simulink model "sampleModel151"  (R2021b)
settings: Solver=VariableStepAuto  StartTime=0.0  StopTime=10.0  RelTol=1e-3
undefined symbols (not defined in the file or in its folder): Newton, Raphson
libraries: simulink x15, slpidlib x2
settings Model: Creator=user  LastModifiedBy=user

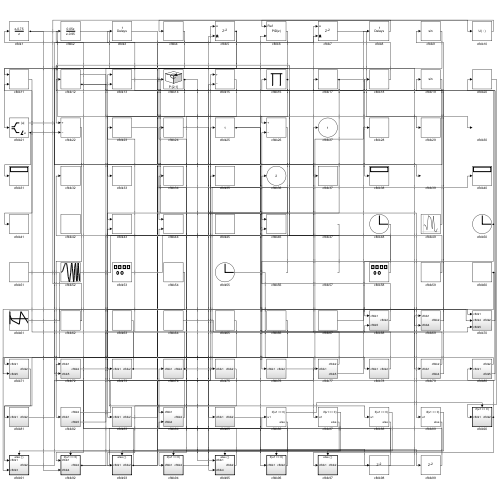
[thumbnail: Simulink's stored preview of the top-level diagram]
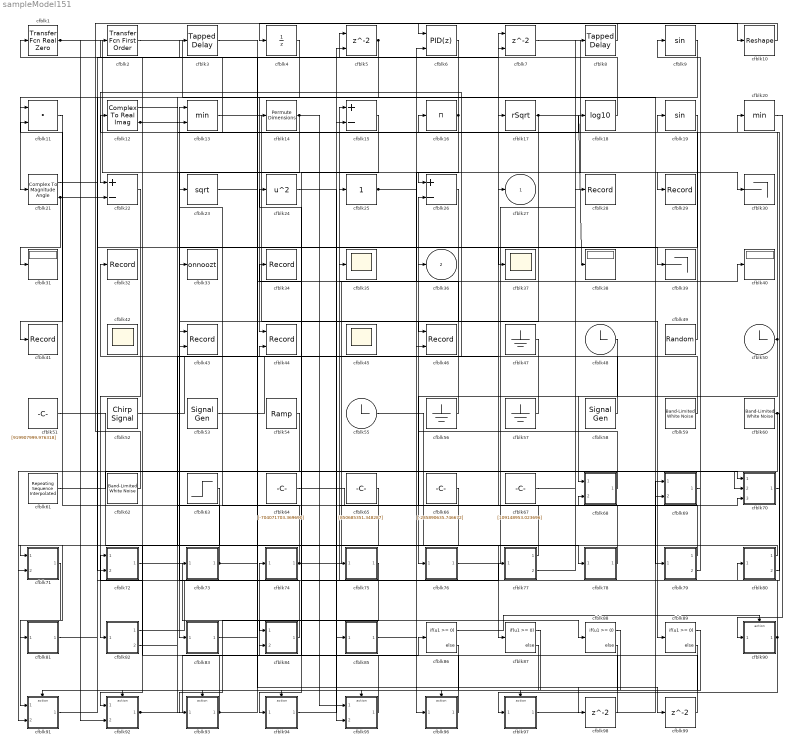
== system sampleModel151 ==
  cfblk1 : simulink/Discrete/Transfer Fcn Real Zero  ZeroZ=0.75  ICPrevInput=0.0  DoSatur=off
      settings: SourceProductBaseCode=SL
  cfblk10 : Reshape
  cfblk11 : DotProduct  InputSameDT=on  OutDataTypeStr=Inherit: Inherit via internal rule
  cfblk12 : ComplexToRealImag
  cfblk13 : MinMax  Inputs=2
  cfblk14 : PermuteDimensions
  cfblk15 : Sum  Inputs=+-
  cfblk16 : Product  Inputs=*
  cfblk17 : Sqrt  Operator=rSqrt  AlgorithmType=Newton-Raphson  SaturateOnIntegerOverflow=on
  cfblk18 : Math  Operator=log10  SaturateOnIntegerOverflow=on
  cfblk19 : Trigonometry
  cfblk2 : simulink/Discrete/Transfer Fcn First Order  PoleZ=0.95  ICPrevOutput=0.0  DoSatur=off
  cfblk20 : MinMax
  cfblk21 : ComplexToMagnitudeAngle
  cfblk22 : Sum  Inputs=+-
  cfblk23 : Sqrt  SaturateOnIntegerOverflow=on
  cfblk24 : Math  Operator=square  SaturateOnIntegerOverflow=on
  cfblk25 : simulink/Math Operations/Slider Gain  gain=1  low=0  high=2
  cfblk26 : Sum  Inputs=+-
  cfblk28 : Record  FileSettingsInternal="{\"entries\":[{\"content\":{\"excelSettings\":{\"content\":{},\"type\":\"Streamout.ExcelSettings\"}},\"type\":\"Streamout.FileSettingStorage\",\"uuid\":\"16329020-b7b2-48e2-bef7-29498af02094\"}],\"packageUris\":[\"http://schema.mathworks.com/mf0/streamout_blocks/R2020a\"],\"version\":\"1.0\"}"  SignalsInternal="{\"entries\":[{\"content\":{\"signals\":[{\"content\":{\"blockPath\":[\"sampleModel151/cfblk28\"],\"channel\":[],\"dimensions\":[1],\"domain\":\"sampleModel151/cfblk28\",\"lineColor\":\"#fe330a\",\"plots\":[1],\"port\":1,\"sid\":[\"\"],\"signalID\":5566,\"signalName\":\"cfblk77:2\"},\"type\":\"RecordBlkView.Signal\",\"uuid\":\"cbec37e1-0653-4d3b-993b-30f071d7b7c2\"}]},\"type\":\"RecordBlkView.InputSignals\",\"uuid\":\"1aea9fb2-e907-4a06-aea3-794993e5d476\"}],\"packageUris\":[\"http://schema.mathworks.com/mf0/streamout_blocks/R2020a\"],\"version\":\"1.0\"}"  VisualizationBindings="{\"sparklinesplugin\":{\"info\":[{\"bindingParametersList\":[],\"subplotID\":1}]}}"
  cfblk29 : Record  FileSettingsInternal="{\"entries\":[{\"content\":{\"excelSettings\":{\"content\":{},\"type\":\"Streamout.ExcelSettings\"}},\"type\":\"Streamout.FileSettingStorage\",\"uuid\":\"ad175cd4-5bed-4ac1-be59-b4bcf34f1e7c\"}],\"packageUris\":[\"http://schema.mathworks.com/mf0/streamout_blocks/R2020a\"],\"version\":\"1.0\"}"  SignalsInternal="{\"entries\":[{\"content\":{\"signals\":[{\"content\":{\"blockPath\":[\"sampleModel151/cfblk29\"],\"channel\":[],\"dimensions\":[1,1],\"domain\":\"sampleModel151/cfblk29\",\"lineColor\":\"#22b573\",\"plots\":[1],\"port\":1,\"sid\":[\"\"],\"signalID\":5570,\"signalName\":\"cfblk7\"},\"type\":\"RecordBlkView.Signal\",\"uuid\":\"59788e8c-d7b2-4cd3-8900-8817d59cbc28\"}]},\"type\":\"RecordBlkView.InputSignals\",\"uuid\":\"d411062e-e278-425d-97f2-c320e6c0c2a0\"}],\"packageUris\":[\"http://schema.mathworks.com/mf0/streamout_blocks/R2020a\"],\"version\":\"1.0\"}"  VisualizationBindings="{\"sparklinesplugin\":{\"info\":[{\"bindingParametersList\":[],\"subplotID\":1}]}}"
  cfblk3 : simulink/Discrete/Tapped Delay  vinit=0.0  samptime=-1  NumDelays=1  DelayOrder=Oldest  includeCurrent=off
  cfblk30 : Terminator
  cfblk31 : Display
  cfblk32 : Record  FileSettingsInternal="{\"entries\":[{\"content\":{\"excelSettings\":{\"content\":{},\"type\":\"Streamout.ExcelSettings\"}},\"type\":\"Streamout.FileSettingStorage\",\"uuid\":\"e17f7bcd-ee65-47d5-ad36-393b5ddf6025\"}],\"packageUris\":[\"http://schema.mathworks.com/mf0/streamout_blocks/R2020a\"],\"version\":\"1.0\"}"  SignalsInternal="{\"entries\":[{\"content\":{\"signals\":[{\"content\":{\"blockPath\":[\"sampleModel151/cfblk32\"],\"channel\":[],\"dimensions\":[1],\"domain\":\"sampleModel151/cfblk32\",\"lineColor\":\"#139fff\",\"plots\":[1],\"port\":1,\"sid\":[\"\"],\"signalID\":5602,\"signalName\":\"cfblk59\"},\"type\":\"RecordBlkView.Signal\",\"uuid\":\"9c12727e-2af6-4ba1-9340-e75212aef403\"}]},\"type\":\"RecordBlkView.InputSignals\",\"uuid\":\"08633602-5334-4035-af5c-359580bce636\"}],\"packageUris\":[\"http://schema.mathworks.com/mf0/streamout_blocks/R2020a\"],\"version\":\"1.0\"}"  VisualizationBindings="{\"sparklinesplugin\":{\"info\":[{\"bindingParametersList\":[],\"subplotID\":1}]}}"
  cfblk33 : ToWorkspace  VariableName=onnoozt  SaveFormat=Timeseries  SampleTime=-1
  cfblk34 : Record  FileSettingsInternal="{\"entries\":[{\"content\":{\"excelSettings\":{\"content\":{},\"type\":\"Streamout.ExcelSettings\"}},\"type\":\"Streamout.FileSettingStorage\",\"uuid\":\"80bf3479-7660-47d1-b758-6739f5e518e5\"}],\"packageUris\":[\"http://schema.mathworks.com/mf0/streamout_blocks/R2020a\"],\"version\":\"1.0\"}"  SignalsInternal="{\"entries\":[{\"content\":{\"signals\":[{\"content\":{\"blockPath\":[\"sampleModel151/cfblk34\"],\"channel\":[],\"dimensions\":[1],\"domain\":\"sampleModel151/cfblk34\",\"lineColor\":\"#0072bd\",\"plots\":[1],\"port\":1,\"sid\":[\"\"],\"signalID\":5574,\"signalName\":\"cfblk90\"},\"type\":\"RecordBlkView.Signal\",\"uuid\":\"52cf2cfa-6272-4b00-98cf-892733082b01\"}]},\"type\":\"RecordBlkView.InputSignals\",\"uuid\":\"b0825b05-81fc-4d9b-a675-fd277561146e\"}],\"packageUris\":[\"http://schema.mathworks.com/mf0/streamout_blocks/R2020a\"],\"version\":\"1.0\"}"  VisualizationBindings="{\"sparklinesplugin\":{\"info\":[{\"bindingParametersList\":[],\"subplotID\":1}]}}"
  cfblk{35,37,42,45} (4 alike) : Scope
      cfblk42 settings: Floating=on
      cfblk45 settings: Floating=on
  cfblk38 : Display
  cfblk39 : Terminator
  cfblk4 : UnitDelay  HasFrameUpgradeWarning=on
  cfblk40 : Display
  cfblk41 : Record  FileSettingsInternal="{\"entries\":[{\"content\":{\"excelSettings\":{\"content\":{},\"type\":\"Streamout.ExcelSettings\"}},\"type\":\"Streamout.FileSettingStorage\",\"uuid\":\"e783f573-5e51-434e-8b39-352c88833e99\"}],\"packageUris\":[\"http://schema.mathworks.com/mf0/streamout_blocks/R2020a\"],\"version\":\"1.0\"}"  SignalsInternal="{\"entries\":[{\"content\":{\"signals\":[{\"content\":{\"blockPath\":[\"sampleModel151/cfblk41\"],\"channel\":[],\"dimensions\":[1],\"domain\":\"sampleModel151/cfblk41\",\"lineColor\":\"#d95319\",\"plots\":[1],\"port\":1,\"sid\":[\"\"],\"signalID\":5578,\"signalName\":\"cfblk11\"},\"type\":\"RecordBlkView.Signal\",\"uuid\":\"9378f9bf-08aa-425a-ab1e-6e49c199abac\"}]},\"type\":\"RecordBlkView.InputSignals\",\"uuid\":\"4020c576-885d-4cd6-9814-44353d409ce4\"}],\"packageUris\":[\"http://schema.mathworks.com/mf0/streamout_blocks/R2020a\"],\"version\":\"1.0\"}"  VisualizationBindings="{\"sparklinesplugin\":{\"info\":[{\"bindingParametersList\":[],\"subplotID\":1}]}}"
  cfblk43 : Record  FileSettingsInternal="{\"entries\":[{\"content\":{\"excelSettings\":{\"content\":{},\"type\":\"Streamout.ExcelSettings\"}},\"type\":\"Streamout.FileSettingStorage\",\"uuid\":\"0c75c6a2-1ebc-4dbd-9707-8aa0bfb7056d\"}],\"packageUris\":[\"http://schema.mathworks.com/mf0/streamout_blocks/R2020a\"],\"version\":\"1.0\"}"  Layout=[1 1]  SignalsInternal="{\"entries\":[{\"content\":{\"signals\":[{\"content\":{\"blockPath\":[\"sampleModel151/cfblk43\"],\"channel\":[],\"dimensions\":[1],\"domain\":\"sampleModel151/cfblk43\",\"lineColor\":\"#a2142f\",\"plots\":[1],\"port\":1,\"sid\":[\"\"],\"signalID\":5582,\"signalName\":\"cfblk26\"},\"type\":\"RecordBlkView.Signal\",\"uuid\":\"05fc9d93-6de0-4f23-9265-e6d9e86d6584\"},{\"content\":{\"blockPath\":[\"sampleModel151/cfblk43\"],\"channel\":[],\"dimensions\":[1],\"domain\":\"sampleModel151/cfblk43\",\"lineColor\":\"#139fff\",\"plots\":[1],\"port\":2,\"sid\":[\"\"],\"signalID\":5606,\"signalName\":\"cfblk47\"},\"type\":\"RecordBlkView.Signal\",\"uuid\":\"81c749a0-ca2e-451c-aa8b-75db0fa4dd54\"}]},\"type\":\"RecordBlkView.InputSignals\",\"uuid\":\"aefd6379-81b4-49ca-99cc-edc691e51c33\"}],\"packageUris\":[\"http://schema.mathworks.com/mf0/streamout_blocks/R2020a\"],\"version\":\"1.0\"}"  VisualizationBindings="{\"xyplotplugin\":{\"info\":[{\"series\":[{\"bindingParametersList\":[{\"parameter\":\"X-Axis\",\"signalID\":5582,\"signalName\":\"cfblk26\"},{\"parameter\":\"Y-Axis\",\"signalID\":5606,\"signalName\":\"cfblk47\"}],\"seriesID\":51947}],\"subplotID\":1}]}}"  CompatibilityTag=XY
  cfblk44 : Record  FileSettingsInternal="{\"entries\":[{\"content\":{\"excelSettings\":{\"content\":{},\"type\":\"Streamout.ExcelSettings\"}},\"type\":\"Streamout.FileSettingStorage\",\"uuid\":\"e408540b-f554-4ccd-875e-bc098b567ff3\"}],\"packageUris\":[\"http://schema.mathworks.com/mf0/streamout_blocks/R2020a\"],\"version\":\"1.0\"}"  Layout=[1 1]  SignalsInternal="{\"entries\":[{\"content\":{\"signals\":[{\"content\":{\"blockPath\":[\"sampleModel151/cfblk44\"],\"channel\":[],\"dimensions\":[1],\"domain\":\"sampleModel151/cfblk44\",\"lineColor\":\"#a2142f\",\"plots\":[1],\"port\":1,\"sid\":[\"\"],\"signalID\":5586,\"signalName\":\"cfblk16\"},\"type\":\"RecordBlkView.Signal\",\"uuid\":\"6af45d05-4fcc-41dc-a0e5-1353e5ef8c24\"},{\"content\":{\"blockPath\":[\"sampleModel151/cfblk44\"],\"channel\":[],\"dimensions\":[1],\"domain\":\"sampleModel151/cfblk44\",\"lineColor\":\"#139fff\",\"plots\":[1],\"port\":2,\"sid\":[\"\"],\"signalID\":5590,\"signalName\":\"cfblk82:2\"},\"type\":\"RecordBlkView.Signal\",\"uuid\":\"fc406fd3-a582-4b99-9ff1-c8c34bae7090\"}]},\"type\":\"RecordBlkView.InputSignals\",\"uuid\":\"f27d2fd3-ba63-49dc-9794-1473fbe6710d\"}],\"packageUris\":[\"http://schema.mathworks.com/mf0/streamout_blocks/R2020a\"],\"version\":\"1.0\"}"  VisualizationBindings="{\"xyplotplugin\":{\"info\":[{\"series\":[{\"bindingParametersList\":[{\"parameter\":\"X-Axis\",\"signalID\":5586,\"signalName\":\"cfblk16\"},{\"parameter\":\"Y-Axis\",\"signalID\":5590,\"signalName\":\"cfblk82:2\"}],\"seriesID\":36672}],\"subplotID\":1}]}}"  CompatibilityTag=XY
  cfblk46 : Record  FileSettingsInternal="{\"entries\":[{\"content\":{\"excelSettings\":{\"content\":{},\"type\":\"Streamout.ExcelSettings\"}},\"type\":\"Streamout.FileSettingStorage\",\"uuid\":\"872aefc3-b221-4a71-9802-efcb06a78721\"}],\"packageUris\":[\"http://schema.mathworks.com/mf0/streamout_blocks/R2020a\"],\"version\":\"1.0\"}"  Layout=[1 1]  SignalsInternal="{\"entries\":[{\"content\":{\"signals\":[{\"content\":{\"blockPath\":[\"sampleModel151/cfblk46\"],\"channel\":[],\"dimensions\":[1],\"domain\":\"sampleModel151/cfblk46\",\"lineColor\":\"#a2142f\",\"plots\":[1],\"port\":1,\"sid\":[\"\"],\"signalID\":5594,\"signalName\":\"cfblk24\"},\"type\":\"RecordBlkView.Signal\",\"uuid\":\"f73d4481-3b9c-43d6-816d-b610603f159a\"},{\"content\":{\"blockPath\":[\"sampleModel151/cfblk46\"],\"channel\":[],\"dimensions\":[1],\"domain\":\"sampleModel151/cfblk46\",\"lineColor\":\"#139fff\",\"plots\":[1],\"port\":2,\"sid\":[\"\"],\"signalID\":5598,\"signalName\":\"cfblk16\"},\"type\":\"RecordBlkView.Signal\",\"uuid\":\"61bf5f49-bdad-4a1e-a78b-57c9270c8f12\"}]},\"type\":\"RecordBlkView.InputSignals\",\"uuid\":\"eca14434-e9e9-4071-bd11-9bcd73b8db11\"}],\"packageUris\":[\"http://schema.mathworks.com/mf0/streamout_blocks/R2020a\"],\"version\":\"1.0\"}"  VisualizationBindings="{\"xyplotplugin\":{\"info\":[{\"series\":[{\"bindingParametersList\":[{\"parameter\":\"X-Axis\",\"signalID\":5594,\"signalName\":\"cfblk24\"},{\"parameter\":\"Y-Axis\",\"signalID\":5598,\"signalName\":\"cfblk16\"}],\"seriesID\":29055}],\"subplotID\":1}]}}"  CompatibilityTag=XY
  cfblk47 : Ground
  cfblk48 : Clock
  cfblk49 : RandomNumber  Mean=[30540.773261]  Variance=[36221.773960]  Seed=[260701924.000000]  SampleTime=0.1
  cfblk5 : Delay  ShowEnablePort=on  SampleTime=1
      settings: InputPortMap=u0,e6
  cfblk50 : Clock
  cfblk51 : Constant  Value=[919907999.976318]  SampleTime=1
  cfblk52 : simulink/Sources/Chirp Signal  f1=[-683339794.347448]  T=[-526882344.998948]  f2=[43752890.467036]
  cfblk53 : SignalGenerator  WaveForm=sawtooth  Amplitude=[-680922363.172468]
  cfblk54 : simulink/Sources/Ramp  slope=[1986.058143]  start=[19.480931]  InitialOutput=[55276.021662]
  cfblk55 : Clock
  cfblk56 : Ground
  cfblk57 : Ground
  cfblk58 : SignalGenerator  WaveForm=sawtooth  Amplitude=[-424760600.039455]
  cfblk59 : simulink/Sources/Band-Limited White Noise  Cov=[1215861451.663982]  Ts=0.1  seed=[1365901163.000000]
  cfblk6 : slpidlib/PID Controller (2DOF)  Controller=PID  Form=Parallel  TimeDomain=Discrete-time  UseExternalTs=off  SampleTime=1  IntegratorMethod=Forward Euler  FilterMethod=Forward Euler  ControllerParametersSource=internal  P=1  I=1  D=0  UseFilter=on  N=100  b=1  c=1  TunerSelectOption=Transfer Function Based (PID Tuner App)  InitialConditionSource=internal  InitialConditionForIntegrator=0  InitialConditionForFilter=0  DifferentiatorICPrevScaledInput=0  ExternalReset=none  TrackingMode=off  Kt=1  LimitOutput=off  SatLimitsSource=internal  UpperSaturationLimit=inf  LowerSaturationLimit=-inf  LinearizeAsGain=off  AntiWindupMode=none  Kb=1  POutMin=[]  POutMax=[]  IOutMin=[]  IOutMax=[]  DOutMin=[]  DOutMax=[]  NOutMin=[]  NOutMax=[]  bOutMin=[]  bOutMax=[]  cOutMin=[]  cOutMax=[]  SumOutMin=[]  SumOutMax=[]  SaturationOutMin=[]  SaturationOutMax=[]  PParamMin=[]  PParamMax=[]  IParamMin=[]  IParamMax=[]  DParamMin=[]  DParamMax=[]  NParamMin=[]  NParamMax=[]  bParamMin=[]  bParamMax=[]  cParamMin=[]  cParamMax=[]  KbParamMin=[]  KbParamMax=[]  KtParamMin=[]  KtParamMax=[]  KbOutMin=[]  KbOutMax=[]  KtOutMin=[]  KtOutMax=[]  IntegratorOutMin=[]  IntegratorOutMax=[]  FilterOutMin=[]  FilterOutMax=[]  SumI1OutMin=[]  SumI1OutMax=[]  SumI2OutMin=[]  SumI2OutMax=[]  SumI3OutMin=[]  SumI3OutMax=[]  SumI4OutMin=[]  SumI4OutMax=[]  SumDOutMin=[]  SumDOutMax=[]  Sum1OutMin=[]  Sum1OutMax=[]  Sum2OutMin=[]  Sum2OutMax=[]  Sum3OutMin=[]  Sum3OutMax=[]  DifferentiatorOutMin=[]  DifferentiatorOutMax=[]  FilterDiffOutCoefMin=[]  FilterDiffOutCoefMax=[]  ReciprocalOutMin=[]  ReciprocalOutMax=[]  SumDenOutMin=[]  SumDenOutMax=[]  SumNumOutMin=[]  SumNumOutMax=[]  DivideOutMin=[]  DivideOutMax=[]  UdiffTsProdOutMin=[]  UdiffTsProdOutMax=[]  NTsProdOutMin=[]  NTsProdOutMax=[]  UintegralTsProdOutMin=[]  UintegralTsProdOutMax=[]  UngainTsProdOutMin=[]  UngainTsProdOutMax=[]  IntegratorContinuousStateAttributes=''  IntegratorStateMustResolveToSignalObject=off  IntegratorRTWStateStorageClass=Auto  FilterContinuousStateAttributes=''  FilterStateMustResolveToSignalObject=off  FilterRTWStateStorageClass=Auto  ParallelPVariant=InternalParameters  IdealPVariant=Disabled  IVariant=InternalParameters  DVariant=InternalParameters  bVariant=InternalParameters  cVariant=InternalParameters  IntegratorVariant=Discrete  SatVariant=Disabled  AWVariant=Passthrough  PCopyVariant=Disabled  TRVariant=Disabled  FdbkBlocksVariant=Forward  IdealPFdbkVariant=Disabled  SatFdbkVariant=Disabled  DerivativeFilterVariant=ForwardEulerFilter  NVariant=InternalParameters  NCopyVariant=Disabled  FilterICVariant=InternalICsFilter  IntegratorICVariant=InternalICs  ExternalResetVariant=Disabled  TRSumVariant=Passthrough  SumFdbkVariant=Disabled  SumVariant=Sum_PID  TsampFilterVariant=InternalTs  TsampNgainVariant=Passthrough  TsampIntegralVariant=Passthrough  ExternalSaturationOutDataTypeStr=Inherit: Same as second input
      settings: SourceProductBaseCode=SL
  cfblk60 : simulink/Sources/Band-Limited White Noise  Cov=[7735132577.981955]  Ts=0.1  seed=[9624433011.000000]
  cfblk61 : simulink/Sources/Repeating Sequence Interpolated  OutValues=[321209929.759004, -164411513.665843, -521363815.949086, 697235986.617966, -429595361.275155]  TimeValues=[0 0.1 0.5 0.6 1].'  LookUpMeth=Use Input Below  tsamp=0.01  OutMin=[]  OutMax=[]  OutDataTypeStr=double  OutputDataTypeScalingMode=double  OutDataType=fixdt(0,8)  OutScaling=2^-10
  cfblk62 : simulink/Sources/Band-Limited White Noise  Cov=[8435027631.011647]  Ts=0.1  seed=[5841098064.000000]
  cfblk63 : Step  Time=[4.000000]  Before=[11276169.714796]  After=[23174660.640238]  SampleTime=0
  cfblk64 : Constant  Value=[-704071703.369690]  SampleTime=1
  cfblk65 : Constant  Value=[850685351.348287]  SampleTime=1
  cfblk66 : Constant  Value=[-285890635.746672]  SampleTime=1
  cfblk67 : Constant  Value=[109148953.023696]  SampleTime=1
  cfblk68 : Subsystem
  cfblk69 : Subsystem
  cfblk7 : Delay  ShowEnablePort=on  SampleTime=1
      settings: InputPortMap=u0,e6
  cfblk70 : Subsystem
  cfblk71 : Subsystem
  cfblk72 : Subsystem
  cfblk73 : Subsystem
  cfblk74 : Subsystem
  cfblk75 : Subsystem
  cfblk76 : Subsystem
  cfblk77 : Subsystem
  cfblk78 : Subsystem
  cfblk79 : Subsystem
  cfblk8 : simulink/Discrete/Tapped Delay  vinit=0.0  samptime=-1  NumDelays=1  DelayOrder=Oldest  includeCurrent=off
  cfblk80 : Subsystem
  cfblk81 : Subsystem
  cfblk82 : Subsystem
  cfblk83 : Subsystem
  cfblk84 : Subsystem
  cfblk85 : Subsystem
  cfblk{86..89} (4 alike) : If  IfExpression=u1 >= 0  SampleTime=1
  cfblk9 : Trigonometry
  cfblk90 : Subsystem  TreatAsAtomicUnit=on
  cfblk91 : Subsystem  TreatAsAtomicUnit=on
  cfblk92 : Subsystem  TreatAsAtomicUnit=on
  cfblk93 : Subsystem  TreatAsAtomicUnit=on
  cfblk94 : Subsystem  TreatAsAtomicUnit=on
  cfblk95 : Subsystem  TreatAsAtomicUnit=on
  cfblk96 : Subsystem  TreatAsAtomicUnit=on
  cfblk97 : Subsystem  TreatAsAtomicUnit=on
  cfblk98 : Delay  SampleTime=1
  cfblk99 : Delay  SampleTime=1
  cfblk27 : Outport
  cfblk36 : Outport  Port=2
  wires:
  cfblk79/1(cfblk2) -> cfblk15/1
  cfblk84/1(cfblk2) -> cfblk13/1
  cfblk16/1 -> cfblk44/1, cfblk46/2
  cfblk92/1(cfblk2) -> cfblk86/1, cfblk70/3(cfblk5)
  cfblk57/1 -> cfblk22/1
  cfblk59/1 -> cfblk32/1
  cfblk85/1(cfblk2) -> cfblk96/1(cfblk1)
  cfblk15/1 -> cfblk94/1(cfblk1)
  cfblk69/1(cfblk2) -> cfblk9/1
  cfblk14/1 -> cfblk83/1(cfblk1), cfblk95/1(cfblk1)
  cfblk80/1(cfblk2) -> cfblk71/1(cfblk1)
  cfblk75/1(cfblk2) -> cfblk93/1(cfblk1)
  cfblk62/1 -> cfblk10/1
  cfblk82/1(cfblk2) -> cfblk25/1
  cfblk22/1 -> cfblk82/1(cfblk1)
  cfblk60/1 -> cfblk80/1(cfblk1), cfblk91/2(cfblk3)
  cfblk65/1 -> cfblk71/2(cfblk5)
  cfblk13/1 -> cfblk89/1
  cfblk93/1(cfblk2) -> cfblk5/1, cfblk40/1, cfblk72/1(cfblk1)
  cfblk77/1(cfblk2) -> cfblk7/1
  cfblk19/1 -> cfblk33/1
  cfblk50/1 -> cfblk68/1(cfblk1), cfblk3/1
  cfblk6/1 -> cfblk21/1
  cfblk9/1 -> cfblk11/1
  cfblk67/1 -> cfblk70/1(cfblk1)
  cfblk66/1 -> cfblk92/1(cfblk1)
  cfblk48/1 -> cfblk76/1(cfblk1)
  cfblk96/1(cfblk2) -> cfblk74/1(cfblk1)
  cfblk1/1 -> cfblk26/1, cfblk92/2(cfblk4)
  cfblk8/1 -> cfblk6/1
  cfblk18/1 -> cfblk1/1
  cfblk20/1 -> cfblk90/1(cfblk1)
  cfblk56/1 -> cfblk35/1
  cfblk90/1(cfblk2) -> cfblk97/1(cfblk1), cfblk34/1
  cfblk53/1 -> cfblk27/1
  cfblk91/1(cfblk2) -> cfblk7/2
  cfblk26/1 -> cfblk43/1
  cfblk21/1 -> cfblk39/1
  cfblk4/1 -> cfblk13/2
  cfblk71/1(cfblk2) -> cfblk91/1(cfblk1)
  cfblk78/1(cfblk2) -> cfblk26/2
  cfblk94/1(cfblk2) -> cfblk5/2
  cfblk55/1 -> cfblk87/1
  cfblk74/1(cfblk2) -> cfblk6/2, cfblk23/1
  cfblk10/1 -> cfblk4/1
  cfblk52/1 -> cfblk15/2
  cfblk80/2(cfblk5) -> cfblk12/1
  cfblk72/1(cfblk2) -> cfblk84/1(cfblk1)
  cfblk12/1 -> cfblk78/1(cfblk1)
  cfblk11/1 -> cfblk41/1
  cfblk97/1(cfblk2) -> cfblk69/1(cfblk1)
  cfblk25/1 -> cfblk69/2(cfblk4), cfblk98/1
  cfblk68/1(cfblk2) -> cfblk36/1
  cfblk24/1 -> cfblk46/1
  cfblk79/2(cfblk4) -> cfblk17/1
  cfblk5/1 -> cfblk22/2, cfblk72/2(cfblk5)
  cfblk2/1 -> cfblk79/1(cfblk1)
  cfblk54/1 -> cfblk73/1(cfblk1)
  cfblk81/1(cfblk2) -> cfblk75/1(cfblk1)
  cfblk64/1 -> cfblk68/2(cfblk5)
  cfblk47/1 -> cfblk43/2
  cfblk49/1 -> cfblk19/1
  cfblk7/1 -> cfblk29/1
  cfblk12/2 -> cfblk30/1, cfblk18/1
  cfblk3/1 -> cfblk88/1
  cfblk58/1 -> cfblk16/1
  cfblk17/1 -> cfblk38/1, cfblk95/2(cfblk4)
  cfblk73/1(cfblk2) -> cfblk14/1, cfblk11/2
  cfblk77/2(cfblk5) -> cfblk28/1
  cfblk76/1(cfblk2) -> cfblk8/1
  cfblk63/1 -> cfblk81/1(cfblk1)
  cfblk51/1 -> cfblk85/1(cfblk1)
  cfblk61/1 -> cfblk70/2(cfblk4)
  cfblk82/2(cfblk5) -> cfblk44/2
  cfblk95/1(cfblk2) -> cfblk24/1
  cfblk21/2 -> cfblk37/1, cfblk31/1
  cfblk70/1(cfblk2) -> cfblk20/1
  cfblk83/1(cfblk2) -> cfblk77/1(cfblk1)
  cfblk86/1 -> cfblk90/Action
  cfblk86/2 -> cfblk91/Action
  cfblk87/1 -> cfblk92/Action
  cfblk87/2 -> cfblk93/Action
  cfblk88/1 -> cfblk94/Action
  cfblk88/2 -> cfblk95/Action
  cfblk89/1 -> cfblk96/Action
  cfblk89/2 -> cfblk97/Action
  cfblk98/1 -> cfblk2/1
  cfblk23/1 -> cfblk99/1
  cfblk99/1 -> cfblk84/2(cfblk4)

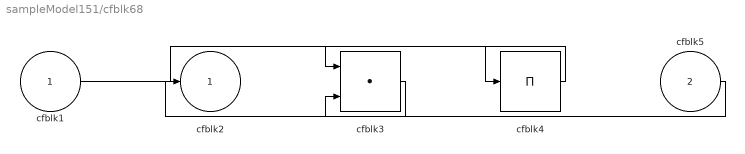
== system sampleModel151/cfblk68 ==
  cfblk1 : Inport
  cfblk5 : Inport  Port=2
  cfblk3 : DotProduct  InputSameDT=on  OutDataTypeStr=Inherit: Inherit via internal rule
  cfblk4 : Product  Inputs=*
  cfblk2 : Outport
  wires:
  cfblk1/1 -> cfblk4/1
  cfblk3/1 -> cfblk2/1
  cfblk4/1 -> cfblk3/1
  cfblk5/1 -> cfblk3/2

== system sampleModel151/cfblk69 ==
  cfblk1 : Inport
  cfblk4 : Inport  Port=2
  cfblk3 : simulink/Discrete/Difference  ICPrevInput=0.0  OutMin=[]  OutMax=[]  OutDataTypeStr=Inherit: Inherit via back propagation  OutDataType=fixdt(1, 16)  OutScaling=2^-10  DoSatur=off
  cfblk2 : Outport
  wires:
  cfblk1/1 -> cfblk3/1
  cfblk4/1 -> cfblk2/1

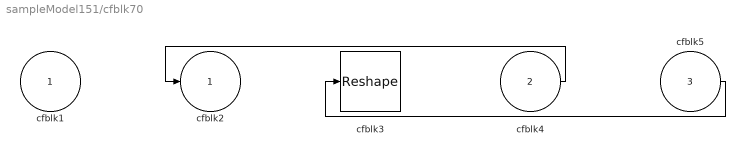
== system sampleModel151/cfblk70 ==
  cfblk1 : Inport
  cfblk4 : Inport  Port=2
  cfblk5 : Inport  Port=3
  cfblk3 : Reshape
  cfblk2 : Outport
  wires:
  cfblk4/1 -> cfblk2/1
  cfblk5/1 -> cfblk3/1

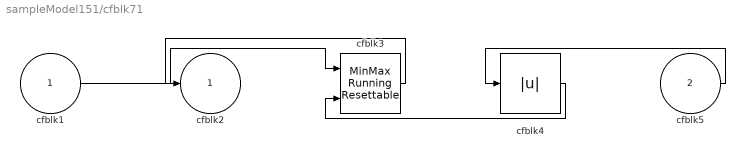
== system sampleModel151/cfblk71 ==
  cfblk1 : Inport
  cfblk5 : Inport  Port=2
  cfblk3 : simulink/Math Operations/MinMax Running Resettable  Function=min  vinit=0.0
  cfblk4 : Abs
  cfblk2 : Outport
  wires:
  cfblk5/1 -> cfblk4/1
  cfblk1/1 -> cfblk3/1
  cfblk4/1 -> cfblk3/2
  cfblk3/1 -> cfblk2/1

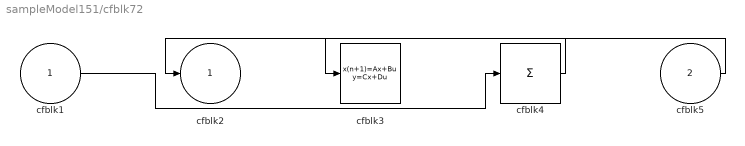
== system sampleModel151/cfblk72 ==
  cfblk1 : Inport
  cfblk5 : Inport  Port=2
  cfblk3 : DiscreteStateSpace
  cfblk4 : Sum  Inputs=+
  cfblk2 : Outport
  wires:
  cfblk5/1 -> cfblk2/1
  cfblk1/1 -> cfblk4/1
  cfblk4/1 -> cfblk3/1

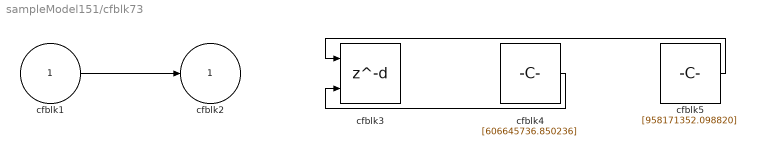
== system sampleModel151/cfblk73 ==
  cfblk1 : Inport
  cfblk3 : Delay  DelayLengthSource=Input port  SampleTime=1
      settings: InputPortMap=u0,p1
  cfblk4 : Constant  Value=[606645736.850236]  SampleTime=1
  cfblk5 : Constant  Value=[958171352.098820]  SampleTime=1
  cfblk2 : Outport
  wires:
  cfblk1/1 -> cfblk2/1
  cfblk5/1 -> cfblk3/1
  cfblk4/1 -> cfblk3/2

== system sampleModel151/cfblk74 ==
  cfblk1 : Inport
  cfblk3 : Sum  Inputs=+
  cfblk4 : Sin  TimeSource=Use external signal  SampleTime=0
  cfblk2 : Outport
  wires:
  cfblk1/1 -> cfblk3/1
  cfblk4/1 -> cfblk2/1
  cfblk3/1 -> cfblk4/1

== system sampleModel151/cfblk75 ==
  cfblk1 : Inport
  cfblk3 : Rounding
  cfblk4 : UnaryMinus
  cfblk2 : Outport
  wires:
  cfblk1/1 -> cfblk4/1
  cfblk4/1 -> cfblk3/1
  cfblk3/1 -> cfblk2/1

== system sampleModel151/cfblk76 ==
  cfblk1 : Inport
  cfblk3 : Constant  Value=[-952970532.415323]  SampleTime=1
  cfblk2 : Outport
  wires:
  cfblk3/1 -> cfblk2/1

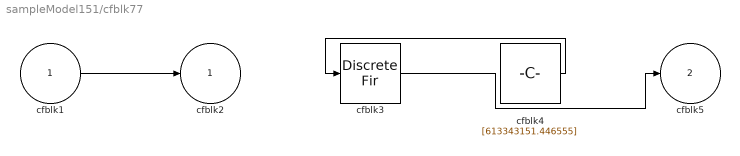
== system sampleModel151/cfblk77 ==
  cfblk1 : Inport
  cfblk3 : DiscreteFir  SampleTime=1
  cfblk4 : Constant  Value=[613343151.446555]  SampleTime=1
  cfblk2 : Outport
  cfblk5 : Outport  Port=2
  wires:
  cfblk4/1 -> cfblk3/1
  cfblk3/1 -> cfblk5/1
  cfblk1/1 -> cfblk2/1

== system sampleModel151/cfblk78 ==
  cfblk1 : Inport
  cfblk3 : DotProduct  InputSameDT=on  OutDataTypeStr=Inherit: Inherit via internal rule
  cfblk2 : Outport
  wires:
  cfblk3/1 -> cfblk2/1
  cfblk1/1 -> cfblk3/1, cfblk3/2

== system sampleModel151/cfblk79 ==
  cfblk1 : Inport
  cfblk3 : DiscreteFir  SampleTime=1
  cfblk2 : Outport
  cfblk4 : Outport  Port=2
  wires:
  cfblk1/1 -> cfblk2/1, cfblk3/1
  cfblk3/1 -> cfblk4/1

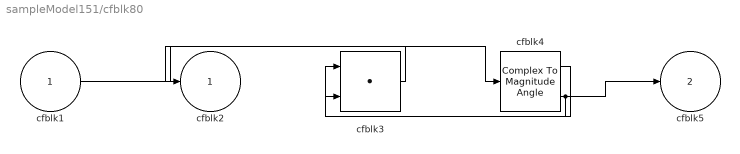
== system sampleModel151/cfblk80 ==
  cfblk1 : Inport
  cfblk3 : DotProduct  InputSameDT=on  OutDataTypeStr=Inherit: Inherit via internal rule
  cfblk4 : ComplexToMagnitudeAngle
  cfblk2 : Outport
  cfblk5 : Outport  Port=2
  wires:
  cfblk1/1 -> cfblk4/1
  cfblk4/1 -> cfblk3/1
  cfblk4/2 -> cfblk3/2, cfblk5/1
  cfblk3/1 -> cfblk2/1

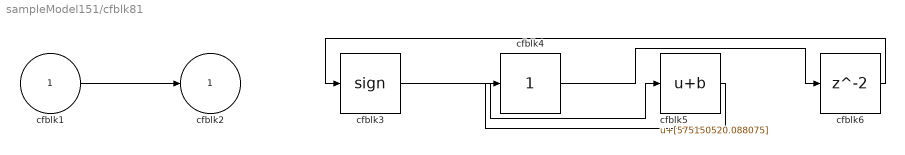
== system sampleModel151/cfblk81 ==
  cfblk1 : Inport
  cfblk3 : Signum
  cfblk4 : simulink/Math Operations/Slider Gain  gain=1  low=0  high=2
  cfblk5 : Bias  Bias=[575150520.088075]
  cfblk6 : Delay  SampleTime=1
  cfblk2 : Outport
  wires:
  cfblk1/1 -> cfblk2/1
  cfblk3/1 -> cfblk5/1
  cfblk5/1 -> cfblk4/1
  cfblk4/1 -> cfblk6/1
  cfblk6/1 -> cfblk3/1

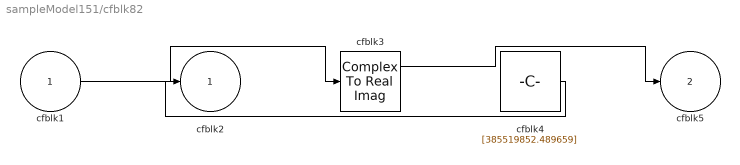
== system sampleModel151/cfblk82 ==
  cfblk1 : Inport
  cfblk3 : ComplexToRealImag
  cfblk4 : Constant  Value=[385519852.489659]  SampleTime=1
  cfblk2 : Outport
  cfblk5 : Outport  Port=2
  wires:
  cfblk1/1 -> cfblk3/1
  cfblk3/1 -> cfblk5/1
  cfblk4/1 -> cfblk2/1

== system sampleModel151/cfblk83 ==
  cfblk1 : Inport
  cfblk3 : Sum  Inputs=+-
  cfblk2 : Outport
  wires:
  cfblk1/1 -> cfblk2/1, cfblk3/1, cfblk3/2

== system sampleModel151/cfblk84 ==
  cfblk1 : Inport
  cfblk4 : Inport  Port=2
  cfblk3 : Abs
  cfblk2 : Outport
  wires:
  cfblk4/1 -> cfblk2/1
  cfblk1/1 -> cfblk3/1

== system sampleModel151/cfblk85 ==
  cfblk1 : Inport
  cfblk3 : slpidlib/PID Controller  Controller=PID  Form=Parallel  TimeDomain=Discrete-time  UseExternalTs=off  SampleTime=1  IntegratorMethod=Forward Euler  FilterMethod=Forward Euler  ControllerParametersSource=internal  P=1  I=1  D=0  UseFilter=on  N=100  TunerSelectOption=Transfer Function Based (PID Tuner App)  InitialConditionSource=internal  InitialConditionForIntegrator=0  InitialConditionForFilter=0  DifferentiatorICPrevScaledInput=0  ExternalReset=none  TrackingMode=off  Kt=1  LimitOutput=off  SatLimitsSource=internal  UpperSaturationLimit=inf  LowerSaturationLimit=-inf  LinearizeAsGain=off  AntiWindupMode=none  Kb=1  POutMin=[]  POutMax=[]  IOutMin=[]  IOutMax=[]  DOutMin=[]  DOutMax=[]  NOutMin=[]  NOutMax=[]  SumOutMin=[]  SumOutMax=[]  SaturationOutMin=[]  SaturationOutMax=[]  PParamMin=[]  PParamMax=[]  IParamMin=[]  IParamMax=[]  DParamMin=[]  DParamMax=[]  NParamMin=[]  NParamMax=[]  KbParamMin=[]  KbParamMax=[]  KtParamMin=[]  KtParamMax=[]  KbOutMin=[]  KbOutMax=[]  KtOutMin=[]  KtOutMax=[]  IntegratorOutMin=[]  IntegratorOutMax=[]  FilterOutMin=[]  FilterOutMax=[]  SumI1OutMin=[]  SumI1OutMax=[]  SumI2OutMin=[]  SumI2OutMax=[]  SumI3OutMin=[]  SumI3OutMax=[]  SumI4OutMin=[]  SumI4OutMax=[]  SumDOutMin=[]  SumDOutMax=[]  DifferentiatorOutMin=[]  DifferentiatorOutMax=[]  FilterDiffOutCoefMin=[]  FilterDiffOutCoefMax=[]  ReciprocalOutMin=[]  ReciprocalOutMax=[]  SumDenOutMin=[]  SumDenOutMax=[]  SumNumOutMin=[]  SumNumOutMax=[]  DivideOutMin=[]  DivideOutMax=[]  UdiffTsProdOutMin=[]  UdiffTsProdOutMax=[]  NTsProdOutMin=[]  NTsProdOutMax=[]  UintegralTsProdOutMin=[]  UintegralTsProdOutMax=[]  UngainTsProdOutMin=[]  UngainTsProdOutMax=[]  IntegratorContinuousStateAttributes=''  IntegratorStateMustResolveToSignalObject=off  IntegratorRTWStateStorageClass=Auto  FilterContinuousStateAttributes=''  FilterStateMustResolveToSignalObject=off  FilterRTWStateStorageClass=Auto  ParallelPVariant=InternalParameters  IdealPVariant=Disabled  IVariant=InternalParameters  DVariant=InternalParameters  IntegratorVariant=Discrete  SatVariant=Disabled  AWVariant=Passthrough  PCopyVariant=Disabled  TRVariant=Disabled  FdbkBlocksVariant=Forward  IdealPFdbkVariant=Disabled  SatFdbkVariant=Disabled  DerivativeFilterVariant=ForwardEulerFilter  NVariant=InternalParameters  NCopyVariant=Disabled  FilterICVariant=InternalICsFilter  IntegratorICVariant=InternalICs  ExternalResetVariant=Disabled  TRSumVariant=Passthrough  SumFdbkVariant=Disabled  SumVariant=Sum_PID  TsampFilterVariant=InternalTs  TsampNgainVariant=Passthrough  TsampIntegralVariant=Passthrough  ExternalSaturationOutDataTypeStr=Inherit: Same as second input
  cfblk4 : Sin  TimeSource=Use external signal  SampleTime=0
  cfblk5 : Delay  SampleTime=1
  cfblk2 : Outport
  wires:
  cfblk1/1 -> cfblk2/1
  cfblk3/1 -> cfblk4/1
  cfblk4/1 -> cfblk5/1
  cfblk5/1 -> cfblk3/1

== system sampleModel151/cfblk90 ==
  cfblk1 : Inport
  Action Port : ActionPort  ActionPortLabel=if(u1 >= 0)
  cfblk3 : DiscreteFir
  cfblk2 : Outport
  wires:
  cfblk1/1 -> cfblk3/1
  cfblk3/1 -> cfblk2/1

== system sampleModel151/cfblk91 ==
  cfblk1 : Inport
  cfblk3 : Inport  Port=2
  Action Port : ActionPort  ActionPortLabel=else
  cfblk2 : Outport
  wires:
  cfblk1/1 -> cfblk2/1

== system sampleModel151/cfblk92 ==
  cfblk1 : Inport
  cfblk4 : Inport  Port=2
  Action Port : ActionPort  ActionPortLabel=if(u1 >= 0)
  cfblk3 : Polyval  Coefs=[ +2.081618890e-019, -1.441693666e-014, +4.719686976e-010, -8.536869453e-006, +1.621573104e-001, -8.087801117e+001 ]
  cfblk2 : Outport
  wires:
  cfblk3/1 -> cfblk2/1
  cfblk1/1 -> cfblk3/1

== system sampleModel151/cfblk93 ==
  cfblk1 : Inport
  Action Port : ActionPort  ActionPortLabel=else
  cfblk3 : Sum  Inputs=|++
  cfblk4 : Constant  Value=[-329229626.774821]  SampleTime=1
  cfblk2 : Outport
  wires:
  cfblk4/1 -> cfblk3/1
  cfblk1/1 -> cfblk3/2
  cfblk3/1 -> cfblk2/1

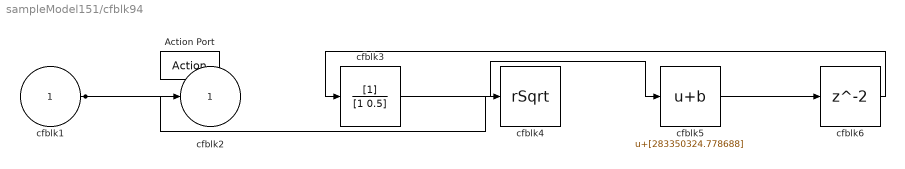
== system sampleModel151/cfblk94 ==
  cfblk1 : Inport
  Action Port : ActionPort  ActionPortLabel=if(u1 >= 0)
  cfblk3 : DiscreteFilter
  cfblk4 : Sqrt  Operator=rSqrt  AlgorithmType=Newton-Raphson  SaturateOnIntegerOverflow=on
  cfblk5 : Bias  Bias=[283350324.778688]
  cfblk6 : Delay
  cfblk2 : Outport
  wires:
  cfblk1/1 -> cfblk2/1, cfblk4/1
  cfblk3/1 -> cfblk5/1
  cfblk5/1 -> cfblk6/1
  cfblk6/1 -> cfblk3/1

== system sampleModel151/cfblk95 ==
  cfblk1 : Inport
  cfblk4 : Inport  Port=2
  Action Port : ActionPort  ActionPortLabel=else
  cfblk3 : Sum  Inputs=+-
  cfblk2 : Outport
  wires:
  cfblk4/1 -> cfblk2/1, cfblk3/2
  cfblk1/1 -> cfblk3/1

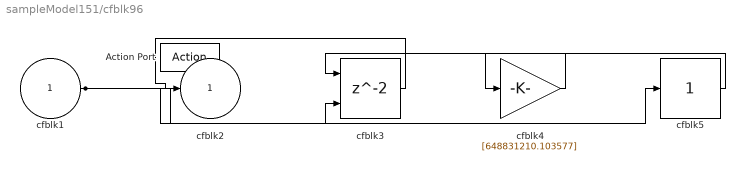
== system sampleModel151/cfblk96 ==
  cfblk1 : Inport
  Action Port : ActionPort  ActionPortLabel=if(u1 >= 0)
  cfblk3 : Delay  ShowEnablePort=on
      settings: InputPortMap=u0,e6
  cfblk4 : Gain  Gain=[648831210.103577]
  cfblk5 : simulink/Math Operations/Slider Gain  gain=1  low=0  high=2
  cfblk2 : Outport
  wires:
  cfblk1/1 -> cfblk5/1, cfblk3/2
  cfblk5/1 -> cfblk4/1
  cfblk3/1 -> cfblk2/1
  cfblk4/1 -> cfblk3/1

== system sampleModel151/cfblk97 ==
  cfblk1 : Inport
  Action Port : ActionPort  ActionPortLabel=else
  cfblk3 : Abs
  cfblk2 : Outport
  wires:
  cfblk1/1 -> cfblk3/1
  cfblk3/1 -> cfblk2/1
